simulink model "SimplePulseGenerator_4x4_HDL_IQ"  (R2019b)
settings: Solver=FixedStepDiscrete  StartTime=0.0  StopTime=inf  RelTol=1e-3
InitFcn:
  | %axis_example_init
  | nco_setup
  | load('iq_bus_obj.mat')
values from neighbouring files (symbols this model uses):
  Fo = 200.7e6    (= 200700000)    [model_init.m]
  Fs = 1/Ts    (= 512000000)    [model_init.m]
  incrScale = (2^N)/Fs    (= 3.2e-05)    [model_init.m]
  N = 14    [model_init.m]
  PRF_count_period = pspshared.libiio.aximm.write(                    'IPAddress',IPAddr,                    'AddressOffset',hex2dec('130'))    [SimplePulseGenerator_4x4_HDL_IQ_IIO_script.m]    (also in model_init.m = 1280)
  PulseWidth_count_width = PulseWidth*fpga_clk_rate/VectorSamplingFactor    (= 32)    [model_init.m]
libraries: hdlsllib x21, simulink x15, dsphdlsigops x4, simulink_need_slupdate x2, dspsrcs4 x1
(part 1 of 2)
Description:
  | HDL model for RFSoC ADC/DAC IQ 8x8 interfacing with the mixer enabled
  | 
  | This model contains demonstrates how to interface to all 8 ADC and 8 DAC
  | channels for the RFSoC.
  | 
  | Please ensure that you run the initialization script to set the correct PLL clock rates.
settings Model: DataTypeOverride=Off  Creator=mfornero  LastModifiedBy=tmealey
settings DataIOCC: SaveOutput=off  SaveTime=off  ReturnWorkspaceOutputs=off
settings OptimizationCC: BlockReduction=off  ConditionallyExecuteInputs=off  DefaultParameterBehavior=Inlined  LifeSpan=inf
settings DebuggingCC: AlgebraicLoopMsg=error  SingleTaskRateTransMsg=error  PregeneratedLibrarySubsystemCodeDiagnostic=none  StrictBusMsg=ErrorOnBusTreatedAsVector  SFUnexpectedBacktrackingDiag=warning  SFNoUnconditionalDefaultTransitionDiag=warning  SFExecutionAtInitializationDiag=none  ArithmeticOperatorsInVariantConditions=warning
settings HardwareCC: ProdBitPerPointer=32  ProdBitPerSizeT=32  ProdBitPerPtrDiffT=32  ProdLargestAtomicFloat=None  ProdIntDivRoundTo=Undefined  ProdEndianess=Unspecified  ProdWordSize=32  ProdHWDeviceType=ASIC/FPGA->ASIC/FPGA  ProdEqTarget=off
settings SFSimCC: SimUseLocalCustomCode=off  CustomCodeUndefinedFunction=UseInterfaceOnly
settings RTWCC: RTWUseLocalCustomCode=off
settings CodeAppCC: StateflowObjectComments=on
settings GRTTargetCC: TargetLangStandard=C89/C90 (ANSI)
settings ConfigComp: CovMetricSettings=dw  CovHtmlReporting=on  CovSaveCumulativeToWorkspaceVar=on  CovSaveSingleToWorkspaceVar=on  CovExternalEMLEnable=off

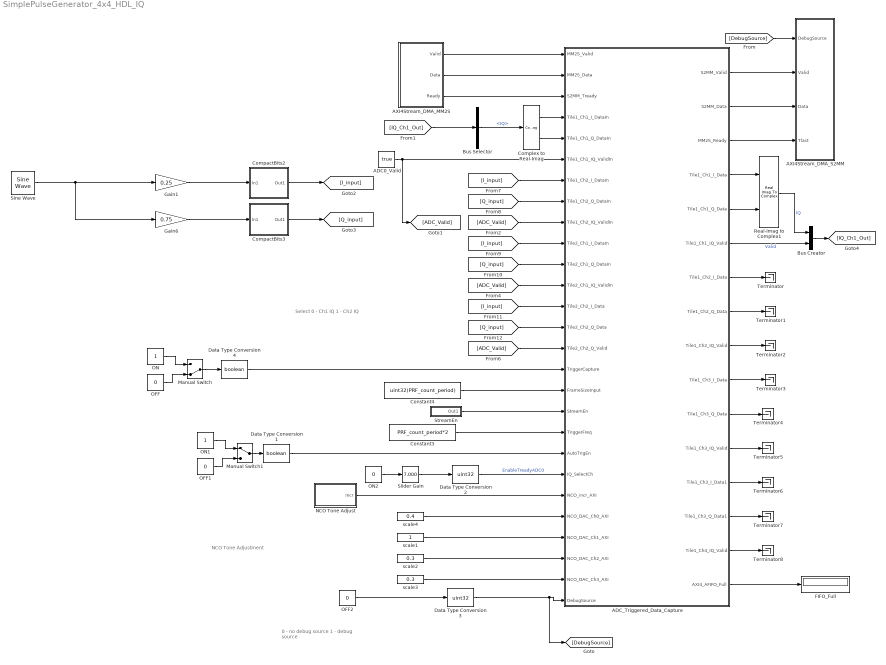
== system SimplePulseGenerator_4x4_HDL_IQ ==
  note: 0 - no debug source
      | 1 - debug source
  note: Select
      |
      | 0 - Ch1 IQ
      | 1 - Ch2 IQ
  note: NCO Tone Adjustment
  ADC0_Valid : Constant  Value=true  SampleTime=-1
  ADC_Triggered_Data_Capture : Subsystem  TreatAsAtomicUnit=on
  AXI4Stream_DMA_MM2S : Subsystem
  AXI4Stream_DMA_S2MM : Subsystem
  Bus Creator : BusCreator  Inputs=2
  Bus Selector : BusSelector  OutputSignals=IQ
  CompactBits2 : Subsystem
  CompactBits3 : Subsystem
  Complex to Real-Imag : ComplexToRealImag
  Constant3 : Constant  Value=PRF_count_period*2  OutDataTypeStr=uint32  SampleTime=-1
  Constant4 : Constant  Value=uint32(PRF_count_period)  SampleTime=-1
  Data Type Conversion1 : DataTypeConversion  OutDataTypeStr=boolean
  Data Type Conversion2 : DataTypeConversion  OutDataTypeStr=uint32
  Data Type Conversion3 : DataTypeConversion  OutDataTypeStr=uint32
  Data Type Conversion4 : DataTypeConversion  OutDataTypeStr=boolean
  FIFO_Full : Display
  Gain1 : Gain  Gain=0.25  OutDataTypeStr=Inherit: Same as input
  Gain6 : Gain  Gain=0.75  OutDataTypeStr=Inherit: Same as input
  Manual Switch : ManualSwitch  CurrentSetting=0
  Manual Switch1 : ManualSwitch
  NCO Tone Adjust : Subsystem
  OFF : Constant  Value=0  OutDataTypeStr=boolean  SampleTime=-1
  OFF1 : Constant  Value=0  OutDataTypeStr=boolean  SampleTime=-1
  OFF2 : Constant  Value=0  OutDataTypeStr=boolean  SampleTime=-1
  ON : Constant  OutDataTypeStr=boolean  SampleTime=-1
  ON1 : Constant  OutDataTypeStr=boolean  SampleTime=-1
  ON2 : Constant  Value=0  OutDataTypeStr=uint32  SampleTime=-1
  Real-Imag to Complex1 : RealImagToComplex
  Sine Wave : dspsrcs4/Sine Wave  Amplitude=1000  Frequency=0.1  Phase=0  SampleMode=Discrete  OutComplex=Real  CompMethod=Table lookup  TableSize=Speed  SampleTime=1/4  SamplesPerFrame=4  ResetState=Restart at time zero  OutputFrames=off  dataType=Fixed-point  wordLen=14  udDataType=sfix(16)  fracBitsMode=User-defined  numFracBits=0  OutDataTypeStr=fixdt(1,14,0)  LastOutDataTypeStr=fixdt(1,14,0)
  Slider Gain : simulink/Math Operations/Slider Gain  gain=7.000  low=0  high=7
  StreamEn : Subsystem
  Terminator{,1..8} (9 alike) : Terminator
  scale1 : Constant  OutDataTypeStr=fixdt(0,8,7)  SampleTime=-1
  scale2 : Constant  Value=0.3  OutDataTypeStr=fixdt(0,8,7)  SampleTime=-1
  scale3 : Constant  Value=0.3  OutDataTypeStr=fixdt(0,8,7)  SampleTime=-1
  scale4 : Constant  Value=0.4  OutDataTypeStr=fixdt(0,8,7)  SampleTime=-1
  wires:
  Data Type Conversion4/1 -> ADC_Triggered_Data_Capture/16(TriggerCapture)
  Constant4/1 -> ADC_Triggered_Data_Capture/17(FrameSizeInput)
  ADC0_Valid/1 -> [ADC_Valid], ADC_Triggered_Data_Capture/6(Tile1_Ch1_IQ_ValidIn)
  Manual Switch/1 -> Data Type Conversion4/1
  ON/1 -> Manual Switch/1
  OFF/1 -> Manual Switch/2
  scale4/1 -> ADC_Triggered_Data_Capture/23(NCO_DAC_Ch0_AXI)
  scale1/1 -> ADC_Triggered_Data_Capture/24(NCO_DAC_Ch1_AXI)
  scale2/1 -> ADC_Triggered_Data_Capture/25(NCO_DAC_Ch2_AXI)
  scale3/1 -> ADC_Triggered_Data_Capture/26(NCO_DAC_Ch3_AXI)
  StreamEn/1(Out1) -> ADC_Triggered_Data_Capture/18(StreamEn)
  Constant3/1 -> ADC_Triggered_Data_Capture/19(TriggerFreq)
  Data Type Conversion1/1 -> ADC_Triggered_Data_Capture/20(AutoTrigEn)
  OFF1/1 -> Manual Switch1/2
  ON1/1 -> Manual Switch1/1
  Manual Switch1/1 -> Data Type Conversion1/1
  ADC_Triggered_Data_Capture/16(AXI4_AFIFO_Full) -> FIFO_Full/1
  ADC_Triggered_Data_Capture/1(S2MM_Valid) -> AXI4Stream_DMA_S2MM/2(Valid)
  ADC_Triggered_Data_Capture/2(S2MM_Data) -> AXI4Stream_DMA_S2MM/3(Data)
  ADC_Triggered_Data_Capture/3(MM2S_Ready) -> AXI4Stream_DMA_S2MM/4(Tlast)
  AXI4Stream_DMA_MM2S/1(Valid) -> ADC_Triggered_Data_Capture/1(MM2S_Valid)
  AXI4Stream_DMA_MM2S/2(Data) -> ADC_Triggered_Data_Capture/2(MM2S_Data)
  AXI4Stream_DMA_MM2S/3(Ready) -> ADC_Triggered_Data_Capture/3(S2MM_Tready)
  ON2/1 -> Slider Gain/1
  Data Type Conversion2/1 -> ADC_Triggered_Data_Capture/21(IQ_SelectCh)  "EnableTreadyADC0"
  NCO Tone Adjust/1(Incr) -> ADC_Triggered_Data_Capture/22(NCO_incr_AXI)
  Slider Gain/1 -> Data Type Conversion2/1
  Sine Wave/1 -> Gain6/1, Gain1/1
  Gain1/1 -> CompactBits2/1(In1)
  Gain6/1 -> CompactBits3/1(In1)
  Data Type Conversion3/1 -> [DebugSource], ADC_Triggered_Data_Capture/27(DebugSource)
  OFF2/1 -> Data Type Conversion3/1
  [DebugSource] -> AXI4Stream_DMA_S2MM/1(DebugSource)
  [ADC_Valid] -> ADC_Triggered_Data_Capture/9(Tile1_Ch2_IQ_ValidIn)
  [ADC_Valid] -> ADC_Triggered_Data_Capture/12(Tile2_Ch1_IQ_ValidIn)
  [ADC_Valid] -> ADC_Triggered_Data_Capture/15(Tile2_Ch2_Q_Valid)
  CompactBits2/1(Out1) -> [I_input]
  CompactBits3/1(Out1) -> [Q_input]
  [I_input] -> ADC_Triggered_Data_Capture/7(Tile1_Ch2_I_DataIn)
  [Q_input] -> ADC_Triggered_Data_Capture/8(Tile1_Ch2_Q_DataIn)
  [I_input] -> ADC_Triggered_Data_Capture/10(Tile2_Ch1_I_DataIn)
  [Q_input] -> ADC_Triggered_Data_Capture/11(Tile2_Ch1_Q_DataIn)
  [I_input] -> ADC_Triggered_Data_Capture/13(Tile2_Ch2_I_Data)
  [Q_input] -> ADC_Triggered_Data_Capture/14(Tile2_Ch2_Q_Data)
  ADC_Triggered_Data_Capture/4(Tile1_Ch1_I_Data) -> Real-Imag to Complex1/1
  ADC_Triggered_Data_Capture/5(Tile1_Ch1_Q_Data) -> Real-Imag to Complex1/2
  Real-Imag to Complex1/1 -> Bus Creator/1  "IQ"
  ADC_Triggered_Data_Capture/6(Tile1_Ch1_IQ_Valid) -> Bus Creator/2  "Valid"
  Bus Creator/1 -> [IQ_Ch1_Out]
  ADC_Triggered_Data_Capture/7(Tile1_Ch2_I_Data) -> Terminator/1
  ADC_Triggered_Data_Capture/8(Tile1_Ch2_Q_Data) -> Terminator1/1
  ADC_Triggered_Data_Capture/9(Tile1_Ch2_IQ_Valid) -> Terminator2/1
  ADC_Triggered_Data_Capture/10(Tile1_Ch3_I_Data) -> Terminator3/1
  ADC_Triggered_Data_Capture/13(Tile1_Ch3_I_Data1) -> Terminator6/1
  ADC_Triggered_Data_Capture/11(Tile1_Ch3_Q_Data) -> Terminator4/1
  ADC_Triggered_Data_Capture/12(Tile1_Ch3_IQ_Valid) -> Terminator5/1
  ADC_Triggered_Data_Capture/14(Tile1_Ch3_Q_Data1) -> Terminator7/1
  ADC_Triggered_Data_Capture/15(Tile1_Ch4_IQ_Valid) -> Terminator8/1
  [IQ_Ch1_Out] -> Bus Selector/1
  Bus Selector/1 -> Complex to Real-Imag/1  "<IQ>"
  Complex to Real-Imag/1 -> ADC_Triggered_Data_Capture/4("Tile1_Ch1_I_DataIn ")
  Complex to Real-Imag/2 -> ADC_Triggered_Data_Capture/5(Tile1_Ch1_Q_DataIn)

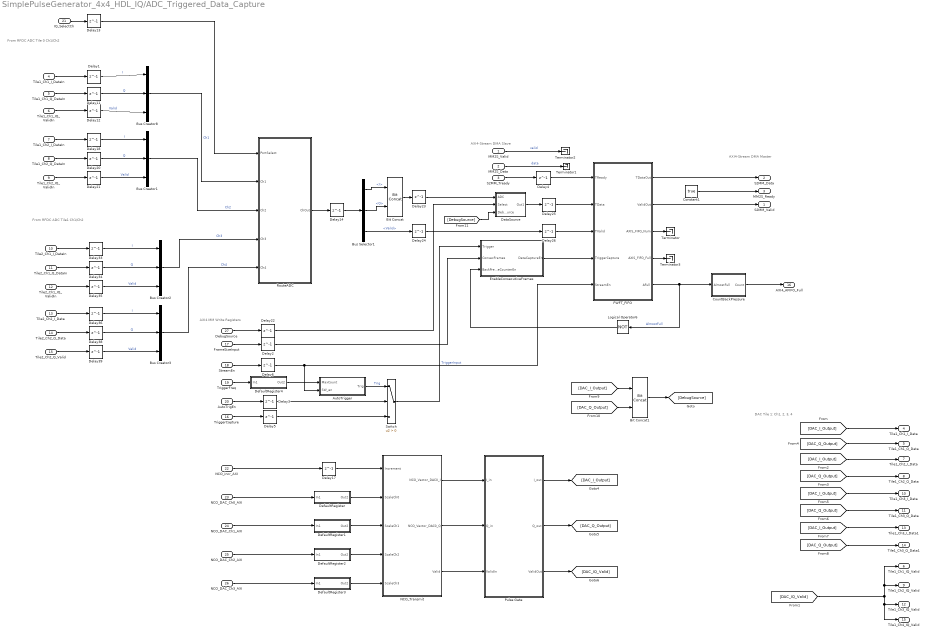
== system SimplePulseGenerator_4x4_HDL_IQ/ADC_Triggered_Data_Capture ==
  note: From RFDC ADC Tile1 Ch1/Ch2
  note: DAC Tile 1: Ch1, 2, 3, 4
  note: AXI4-Stream DMA Slave
  note: AXI4-Stream DMA Master
  note: AXI4 MM Write Registers
  note: From RFDC ADC Tile 0 Ch1/Ch2
  MM2S_Valid : Inport
  MM2S_Data : Inport  Port=2
  S2MM_Tready : Inport  Port=3
  "Tile1_Ch1_I_DataIn " : Inport  Port=4
  Tile1_Ch1_Q_DataIn : Inport  Port=5
  Tile1_Ch1_IQ_ValidIn : Inport  Port=6
  Tile1_Ch2_I_DataIn : Inport  Port=7
  Tile1_Ch2_Q_DataIn : Inport  Port=8
  Tile1_Ch2_IQ_ValidIn : Inport  Port=9
  Tile2_Ch1_I_DataIn : Inport  Port=10
  Tile2_Ch1_Q_DataIn : Inport  Port=11
  Tile2_Ch1_IQ_ValidIn : Inport  Port=12
  Tile2_Ch2_I_Data : Inport  Port=13
  Tile2_Ch2_Q_Data : Inport  Port=14
  Tile2_Ch2_Q_Valid : Inport  Port=15
  TriggerCapture : Inport  Port=16
  FrameSizeInput : Inport  Port=17
  StreamEn : Inport  Port=18
  TriggerFreq : Inport  Port=19
  AutoTrigEn : Inport  Port=20
  IQ_SelectCh : Inport  Port=21
  NCO_incr_AXI : Inport  Port=22
  NCO_DAC_Ch0_AXI : Inport  Port=23
  NCO_DAC_Ch1_AXI : Inport  Port=24
  NCO_DAC_Ch2_AXI : Inport  Port=25
  NCO_DAC_Ch3_AXI : Inport  Port=26
  DebugSource : Inport  Port=27
  AutoTrigger : Subsystem
  Bit Concat : hdlsllib/Logic and Bit Operations/Bit Concat  numInputs=2
      settings: SourceProductName=HDL Coder  SourceProductBaseCode=HD
  Bit Concat1 : hdlsllib/Logic and Bit Operations/Bit Concat  numInputs=2
      settings: SourceProductName=HDL Coder  SourceProductBaseCode=HD
  Bus Creator{1..3,8} (4 alike) : BusCreator  Inputs=3
  Bus Selector1 : BusSelector  OutputSignals=I,Q,Valid
  Constant1 : Constant  Value=true  OutDataTypeStr=boolean  SampleTime=-1
  CountBackPressure : Subsystem
  DataSource : Subsystem
  DefaultRegister : Subsystem
  DefaultRegister1 : Subsystem
  DefaultRegister2 : Subsystem
  DefaultRegister3 : Subsystem
  DefaultRegister4 : Subsystem
  Delay{1..6,11..14,17..18,20..26,33..36,38..39} (25 alike) : Delay  DelayLength=1
  EnableConsecutiveFrames : Subsystem
  FWFT_FIFO : Subsystem
  Logical Operator6 : Logic  Operator=NOT  IconShape=distinctive  AllPortsSameDT=off  OutDataTypeStr=boolean
  NCO_Transmit : Subsystem
  Pulse Gate : Subsystem
      settings: PortSchema="{\"entries\":[{\"content\":{\"sides\":[{\"content\":{\"connectorIds\":[\"In1\",\"In2\",\"In3\"]},\"type\":\"ConnectorPlacement.EquallySpacedRectSide\",\"uuid\":\"05cb44ea-d8d3-4536-b0b5-e0a95c346195\"},{\"content\":{\"connectorIds\":[\"Out1\",\"Out2\",\"Out3\"],\"side\":\"RIGHT\"},\"type\":\"ConnectorPlacement.EquallySpacedRectSide\",\"uuid\":\"95be599f-089a-458f-a20e-438c80ac73ea\"},{\"content\":{\"connectorIds\":[],\"side\":\"TOP\"},\"type\":\"ConnectorPlacement.EquallySpacedRectSide\",\"uuid\":\"53fe8b3e-6af9-4ca4-9119-803948436d03\"}]},\"type\":\"ConnectorPlacement.EquallySpacedConnector\",\"uuid\":\"f0d860a0-0621-4618-986c-a12bc105ad67\"}],\"packageUris\":[\"http://schema.mathworks.com/mf0/Connector/19700101\"],\"version\":\"1.0\"}"
  RouteADC : Subsystem
  Switch : Switch  Criteria=u2 > Threshold
  Terminator{,1..3} (4 alike) : Terminator
  S2MM_Valid : Outport  VectorParamsAs1DForOutWhenUnconnected=off
  S2MM_Data : Outport  Port=2  VectorParamsAs1DForOutWhenUnconnected=off
  MM2S_Ready : Outport  Port=3  VectorParamsAs1DForOutWhenUnconnected=off
  Tile1_Ch1_I_Data : Outport  Port=4  VectorParamsAs1DForOutWhenUnconnected=off
  Tile1_Ch1_Q_Data : Outport  Port=5  VectorParamsAs1DForOutWhenUnconnected=off
  Tile1_Ch1_IQ_Valid : Outport  Port=6  VectorParamsAs1DForOutWhenUnconnected=off
  Tile1_Ch2_I_Data : Outport  Port=7  VectorParamsAs1DForOutWhenUnconnected=off
  Tile1_Ch2_Q_Data : Outport  Port=8  VectorParamsAs1DForOutWhenUnconnected=off
  Tile1_Ch2_IQ_Valid : Outport  Port=9  VectorParamsAs1DForOutWhenUnconnected=off
  Tile1_Ch3_I_Data : Outport  Port=10  VectorParamsAs1DForOutWhenUnconnected=off
  Tile1_Ch3_Q_Data : Outport  Port=11  VectorParamsAs1DForOutWhenUnconnected=off
  Tile1_Ch3_IQ_Valid : Outport  Port=12  VectorParamsAs1DForOutWhenUnconnected=off
  Tile1_Ch3_I_Data1 : Outport  Port=13  VectorParamsAs1DForOutWhenUnconnected=off
  Tile1_Ch3_Q_Data1 : Outport  Port=14  VectorParamsAs1DForOutWhenUnconnected=off
  Tile1_Ch4_IQ_Valid : Outport  Port=15  VectorParamsAs1DForOutWhenUnconnected=off
  AXI4_AFIFO_Full : Outport  Port=16  VectorParamsAs1DForOutWhenUnconnected=off
  wires:
  MM2S_Valid/1 -> Terminator2/1  "valid"
  "Tile1_Ch1_I_DataIn "/1 -> Delay1/1
  MM2S_Data/1 -> Terminator1/1  "data"
  FWFT_FIFO/1(TDataOut) -> S2MM_Data/1
  FrameSizeInput/1 -> Delay2/1
  TriggerCapture/1 -> Delay5/1
  Delay5/1 -> Switch/3
  Delay2/1 -> EnableConsecutiveFrames/2(ConsecFrames)
  S2MM_Tready/1 -> Delay4/1
  Delay4/1 -> FWFT_FIFO/1(TReady)
  StreamEn/1 -> Delay6/1
  Delay6/1 -> AutoTrigger/2(SW_en), FWFT_FIFO/5(StreamEn)
  FWFT_FIFO/2(ValidOut) -> S2MM_Valid/1
  Constant1/1 -> MM2S_Ready/1
  NCO_incr_AXI/1 -> Delay17/1
  NCO_DAC_Ch0_AXI/1 -> DefaultRegister/1(In1)
  Delay17/1 -> NCO_Transmit/1(Increment)
  DefaultRegister/1(Out2) -> NCO_Transmit/2(ScaleCh0)
  DefaultRegister1/1(Out2) -> NCO_Transmit/3(ScaleCh1)
  DefaultRegister2/1(Out2) -> NCO_Transmit/4(ScaleCh2)
  DefaultRegister3/1(Out2) -> NCO_Transmit/5(ScaleCh3)
  NCO_DAC_Ch1_AXI/1 -> DefaultRegister1/1(In1)
  NCO_DAC_Ch2_AXI/1 -> DefaultRegister2/1(In1)
  NCO_DAC_Ch3_AXI/1 -> DefaultRegister3/1(In1)
  FWFT_FIFO/5(AFull) -> CountBackPressure/1(AlmostFull), Logical Operator6/1  "AlmostFull"
  Logical Operator6/1 -> EnableConsecutiveFrames/3(BackPressureCounterEn)
  EnableConsecutiveFrames/1(DataCaptureEn) -> FWFT_FIFO/4(TriggerCapture)
  Switch/1 -> EnableConsecutiveFrames/1(Trigger)  "TriggerInput"
  AutoTrigger/1(Trig) -> Switch/1  "Trig"
  TriggerFreq/1 -> DefaultRegister4/1(In1)
  DefaultRegister4/1(Out2) -> AutoTrigger/1(MaxCount)
  AutoTrigEn/1 -> Delay3/1
  Tile1_Ch1_IQ_ValidIn/1 -> Delay12/1
  Tile1_Ch1_Q_DataIn/1 -> Delay11/1
  Bus Selector1/3 -> Delay24/1  "<Valid>"
  IQ_SelectCh/1 -> Delay13/1
  Delay14/1 -> Bus Selector1/1
  Tile1_Ch2_I_DataIn/1 -> Delay18/1
  Tile1_Ch2_Q_DataIn/1 -> Delay20/1
  Tile1_Ch2_IQ_ValidIn/1 -> Delay21/1
  RouteADC/1(ChOut) -> Delay14/1
  Delay13/1 -> RouteADC/1(PortSelect)
  Bus Selector1/1 -> Bit Concat/1  "<I>"
  Bus Selector1/2 -> Bit Concat/2  "<Q>"
  Bit Concat/1 -> Delay23/1
  DebugSource/1 -> Delay22/1
  Delay24/1 -> Delay26/1
  Delay25/1 -> FWFT_FIFO/2(TData)
  Delay26/1 -> FWFT_FIFO/3(TValid)
  Delay23/1 -> DataSource/1(ADC)
  Delay22/1 -> DataSource/2(Select)
  DataSource/1(Out1) -> Delay25/1
  [DAC_IQ_Valid] -> Tile1_Ch1_IQ_Valid/1, Tile1_Ch2_IQ_Valid/1, Tile1_Ch4_IQ_Valid/1, Tile1_Ch3_IQ_Valid/1
  Tile2_Ch2_Q_Data/1 -> Delay38/1
  Delay39/1 -> Bus Creator3/3  "Valid"
  Tile2_Ch2_I_Data/1 -> Delay36/1
  Delay35/1 -> Bus Creator2/3  "Valid"
  Tile2_Ch1_Q_DataIn/1 -> Delay34/1
  Delay38/1 -> Bus Creator3/2  "Q"
  Tile2_Ch2_Q_Valid/1 -> Delay39/1
  Delay36/1 -> Bus Creator3/1  "I"
  Tile2_Ch1_IQ_ValidIn/1 -> Delay35/1
  Delay33/1 -> Bus Creator2/1  "I"
  Tile2_Ch1_I_DataIn/1 -> Delay33/1
  Delay34/1 -> Bus Creator2/2  "Q"
  Bus Creator2/1 -> RouteADC/4(Ch3)  "Ch3"
  Bus Creator8/1 -> RouteADC/2(Ch1)  "Ch1"
  FWFT_FIFO/3(AXIS_FIFO_Num) -> Terminator/1
  FWFT_FIFO/4(AXIS_FIFO_Full) -> Terminator3/1
  CountBackPressure/1(Count) -> AXI4_AFIFO_Full/1
  Delay11/1 -> Bus Creator8/2  "Q"
  Delay1/1 -> Bus Creator8/1  "I"
  Delay12/1 -> Bus Creator8/3  "Valid"
  Delay18/1 -> Bus Creator1/1  "I"
  Delay20/1 -> Bus Creator1/2  "Q"
  Delay21/1 -> Bus Creator1/3  "Valid"
  Bus Creator1/1 -> RouteADC/3(Ch2)  "Ch2"
  Bus Creator3/1 -> RouteADC/5(Ch4)  "Ch4"
  [DAC_I_Output] -> Tile1_Ch1_I_Data/1
  [DAC_I_Output] -> Tile1_Ch2_I_Data/1
  [DAC_Q_Output] -> Tile1_Ch1_Q_Data/1
  [DAC_Q_Output] -> Tile1_Ch2_Q_Data/1
  [DAC_I_Output] -> Tile1_Ch3_I_Data/1
  [DAC_Q_Output] -> Tile1_Ch3_Q_Data/1
  [DAC_Q_Output] -> Tile1_Ch3_Q_Data1/1
  [DAC_I_Output] -> Tile1_Ch3_I_Data1/1
  Delay3/1 -> Switch/2
  NCO_Transmit/3(Valid) -> Pulse Gate/3(ValidIn)
  NCO_Transmit/1(NCO_Vector_DAC0_I) -> Pulse Gate/1(I_in)
  NCO_Transmit/2(NCO_Vector_DAC0_Q) -> Pulse Gate/2(Q_in)
  Pulse Gate/1(I_out) -> [DAC_I_Output]
  Pulse Gate/2(Q_out) -> [DAC_Q_Output]
  Pulse Gate/3(ValidOut) -> [DAC_IQ_Valid]
  [DAC_I_Output] -> Bit Concat1/1
  [DAC_Q_Output] -> Bit Concat1/2
  Bit Concat1/1 -> [DebugSource]
  [DebugSource] -> DataSource/3(DebugSource)

== system SimplePulseGenerator_4x4_HDL_IQ/AXI4Stream_DMA_MM2S ==
  Constant : Constant  Value=true  SampleTime=-1
  S2MM DMA Ready : Constant  Value=true  SampleTime=-1
  TData : Constant  Value=0  OutDataTypeStr=fixdt(0,128,0)  SampleTime=-1
  Valid : Outport  VectorParamsAs1DForOutWhenUnconnected=off
  Data : Outport  Port=2  VectorParamsAs1DForOutWhenUnconnected=off
  Ready : Outport  Port=3  VectorParamsAs1DForOutWhenUnconnected=off
  wires:
  S2MM DMA Ready/1 -> Ready/1
  TData/1 -> Data/1
  Constant/1 -> Valid/1

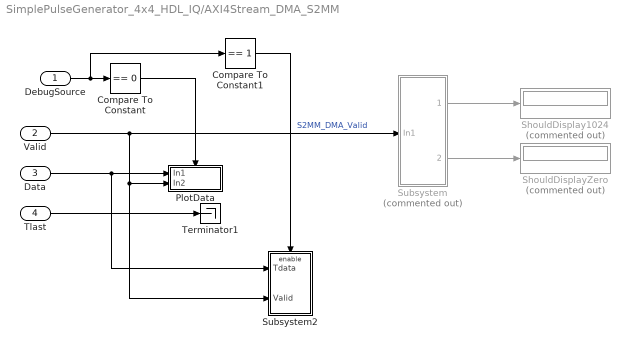
== system SimplePulseGenerator_4x4_HDL_IQ/AXI4Stream_DMA_S2MM ==
  DebugSource : Inport
  Valid : Inport  Port=2
  Data : Inport  Port=3
  Tlast : Inport  Port=4
  Compare To Constant : simulink/Logic and Bit Operations/Compare To Constant  relop===  const=0  OutDataTypeStr=boolean
  Compare To Constant1 : simulink/Logic and Bit Operations/Compare To Constant  relop===  const=1  OutDataTypeStr=boolean
  PlotData : Subsystem
  ShouldDisplay1024 : Display  Commented=on
  ShouldDisplayZero : Display  Commented=on
  Subsystem : Subsystem  Commented=on
  Subsystem2 : Subsystem
  Terminator1 : Terminator
  wires:
  Tlast/1 -> Terminator1/1
  Subsystem/1(Out1) -> ShouldDisplay1024/1
  Subsystem/2(Out2) -> ShouldDisplayZero/1
  Valid/1 -> Subsystem2/2(Valid), PlotData/2(In2), Subsystem/1(In1)  "S2MM_DMA_Valid"
  Data/1 -> Subsystem2/1(Tdata), PlotData/1(In1)
  DebugSource/1 -> Compare To Constant1/1, Compare To Constant/1
  Compare To Constant/1 -> PlotData/Enable
  Compare To Constant1/1 -> Subsystem2/Enable

== system SimplePulseGenerator_4x4_HDL_IQ/CompactBits2 ==
  In1 : Inport
  Bit Concat : hdlsllib/Logic and Bit Operations/Bit Concat  numInputs=4
      settings: SourceProductName=HDL Coder  SourceProductBaseCode=HD
  Data Type Conversion{,1..3} (4 alike) : DataTypeConversion  OutDataTypeStr=fixdt(1,16,0)  ConvertRealWorld=Stored Integer (SI)
  Demux : Demux
  Out1 : Outport  VectorParamsAs1DForOutWhenUnconnected=off
  wires:
  Demux/4 -> Data Type Conversion3/1
  Demux/1 -> Data Type Conversion/1
  Data Type Conversion3/1 -> Bit Concat/1
  Demux/2 -> Data Type Conversion1/1
  Data Type Conversion2/1 -> Bit Concat/2
  Bit Concat/1 -> Out1/1
  Data Type Conversion/1 -> Bit Concat/4
  Data Type Conversion1/1 -> Bit Concat/3
  Demux/3 -> Data Type Conversion2/1
  In1/1 -> Demux/1

== system SimplePulseGenerator_4x4_HDL_IQ/CompactBits3 ==
  In1 : Inport
  Bit Concat : hdlsllib/Logic and Bit Operations/Bit Concat  numInputs=4
      settings: SourceProductName=HDL Coder  SourceProductBaseCode=HD
  Data Type Conversion{,1..3} (4 alike) : DataTypeConversion  OutDataTypeStr=fixdt(1,16,0)  ConvertRealWorld=Stored Integer (SI)
  Demux : Demux
  Out1 : Outport  VectorParamsAs1DForOutWhenUnconnected=off
  wires:
  In1/1 -> Demux/1
  Demux/3 -> Data Type Conversion2/1
  Data Type Conversion1/1 -> Bit Concat/3
  Data Type Conversion/1 -> Bit Concat/4
  Bit Concat/1 -> Out1/1
  Data Type Conversion2/1 -> Bit Concat/2
  Demux/2 -> Data Type Conversion1/1
  Data Type Conversion3/1 -> Bit Concat/1
  Demux/1 -> Data Type Conversion/1
  Demux/4 -> Data Type Conversion3/1

== system SimplePulseGenerator_4x4_HDL_IQ/NCO Tone Adjust ==
  Constant2 : Constant  SampleTime=-1
  Data Type Conversion : DataTypeConversion  OutDataTypeStr=uint16
  Freq (MHz) : simulink/Math Operations/Slider Gain  gain=57.5  low=0  high=250
  Gain : Gain  Gain=1e6
  Gain1 : Gain  Gain=incrScale
  Incr : Outport  VectorParamsAs1DForOutWhenUnconnected=off
  wires:
  Freq (MHz)/1 -> Gain/1
  Constant2/1 -> Freq (MHz)/1
  Data Type Conversion/1 -> Incr/1
  Gain1/1 -> Data Type Conversion/1
  Gain/1 -> Gain1/1

== system SimplePulseGenerator_4x4_HDL_IQ/StreamEn ==
  Data Type Conversion1 : DataTypeConversion  OutDataTypeStr=boolean
  Manual Switch1 : ManualSwitch
  OFF1 : Constant  Value=0  OutDataTypeStr=boolean  SampleTime=-1
  ON1 : Constant  OutDataTypeStr=boolean  SampleTime=-1
  Out1 : Outport  VectorParamsAs1DForOutWhenUnconnected=off
  wires:
  Data Type Conversion1/1 -> Out1/1
  OFF1/1 -> Manual Switch1/2
  ON1/1 -> Manual Switch1/1
  Manual Switch1/1 -> Data Type Conversion1/1

== system SimplePulseGenerator_4x4_HDL_IQ/ADC_Triggered_Data_Capture/AutoTrigger ==
  MaxCount : Inport
  SW_en : Inport  Port=2
  DataPushFrequency : hdlsllib/Sources/HDL Counter  CountType=Free running  CountInit=0  CountStep=1  CountMax=25  CountFromType=Initial value  CountFrom=0  CountResetPort=on  CountLoadPort=off  CountEnbPort=on  CountDirPort=off  CountDataType=Unsigned  CountWordLen=32  CountFracLen=0  CountSampTime=1
      settings: SourceProductBaseCode=HD
  Detect Increase : simulink/Logic and Bit Operations/Detect Increase  vinit=0.0  OutDataTypeStr=boolean
  Relational Operator : RelationalOperator  Operator===  OutDataTypeStr=boolean  RndMeth=Simplest
  Trig : Outport  VectorParamsAs1DForOutWhenUnconnected=off
  wires:
  Relational Operator/1 -> DataPushFrequency/1, Detect Increase/1
  DataPushFrequency/1 -> Relational Operator/2  "DataPushFrequencyCount"
  Detect Increase/1 -> Trig/1
  SW_en/1 -> DataPushFrequency/2
  MaxCount/1 -> Relational Operator/1

== system SimplePulseGenerator_4x4_HDL_IQ/ADC_Triggered_Data_Capture/CountBackPressure ==
  AlmostFull : Inport
  Add : Sum  AccumDataTypeStr=uint32
  Data Type Conversion : DataTypeConversion  OutDataTypeStr=uint32
  Delay16 : Delay  DelayLength=1
  Count : Outport  VectorParamsAs1DForOutWhenUnconnected=off
  wires:
  Delay16/1 -> Count/1, Add/2
  Add/1 -> Delay16/1
  Data Type Conversion/1 -> Add/1
  AlmostFull/1 -> Data Type Conversion/1

== system SimplePulseGenerator_4x4_HDL_IQ/ADC_Triggered_Data_Capture/DataSource ==
  ADC : Inport
  Select : Inport  Port=2
  DebugSource : Inport  Port=3
  Multiport Switch : MultiPortSwitch  DataPortOrder=Zero-based contiguous  Inputs=2  DataPortForDefault=Additional data port  DiagnosticForDefault=Warning  zeroidx=on
  Out1 : Outport  VectorParamsAs1DForOutWhenUnconnected=off
  wires:
  ADC/1 -> Multiport Switch/2, Multiport Switch/4
  Select/1 -> Multiport Switch/1
  DebugSource/1 -> Multiport Switch/3
  Multiport Switch/1 -> Out1/1

== system SimplePulseGenerator_4x4_HDL_IQ/ADC_Triggered_Data_Capture/DefaultRegister ==
  note: Give it default non-zero value at start-up time
  In1 : Inport
  Compare To Zero : simulink/Logic and Bit Operations/Compare To Zero  relop===  OutDataTypeStr=boolean
  Constant5 : Constant  Value=0.0625  OutDataTypeStr=fixdt(0,4,4)  SampleTime=-1
  Delay1 : Delay  DelayLength=1
  Switch2 : Switch  Criteria=u2 > Threshold
  Out2 : Outport  VectorParamsAs1DForOutWhenUnconnected=off
  wires:
  In1/1 -> Delay1/1
  Constant5/1 -> Switch2/1
  Delay1/1 -> Switch2/3, Compare To Zero/1
  Switch2/1 -> Out2/1
  Compare To Zero/1 -> Switch2/2

== system SimplePulseGenerator_4x4_HDL_IQ/ADC_Triggered_Data_Capture/DefaultRegister1 ==
  note: Give it default non-zero value at start-up time
  In1 : Inport
  Compare To Zero : simulink/Logic and Bit Operations/Compare To Zero  relop===  OutDataTypeStr=boolean
  Constant5 : Constant  Value=0.3  OutDataTypeStr=fixdt(0,4,4)  SampleTime=-1
  Delay1 : Delay  DelayLength=1
  Switch2 : Switch  Criteria=u2 > Threshold
  Out2 : Outport  VectorParamsAs1DForOutWhenUnconnected=off
  wires:
  Compare To Zero/1 -> Switch2/2
  Switch2/1 -> Out2/1
  Delay1/1 -> Compare To Zero/1, Switch2/3
  Constant5/1 -> Switch2/1
  In1/1 -> Delay1/1

== system SimplePulseGenerator_4x4_HDL_IQ/ADC_Triggered_Data_Capture/DefaultRegister2 ==
  note: Give it default non-zero value at start-up time
  In1 : Inport
  Compare To Zero : simulink/Logic and Bit Operations/Compare To Zero  relop===  OutDataTypeStr=boolean
  Constant5 : Constant  Value=0.3  OutDataTypeStr=fixdt(0,4,4)  SampleTime=-1
  Delay1 : Delay  DelayLength=1
  Switch2 : Switch  Criteria=u2 > Threshold
  Out2 : Outport  VectorParamsAs1DForOutWhenUnconnected=off
  wires:
  In1/1 -> Delay1/1
  Constant5/1 -> Switch2/1
  Delay1/1 -> Switch2/3, Compare To Zero/1
  Switch2/1 -> Out2/1
  Compare To Zero/1 -> Switch2/2

== system SimplePulseGenerator_4x4_HDL_IQ/ADC_Triggered_Data_Capture/DefaultRegister3 ==
  note: Give it default non-zero value at start-up time
  In1 : Inport
  Compare To Zero : simulink/Logic and Bit Operations/Compare To Zero  relop===  OutDataTypeStr=boolean
  Constant5 : Constant  Value=0.3  OutDataTypeStr=fixdt(0,4,4)  SampleTime=-1
  Delay1 : Delay  DelayLength=1
  Switch2 : Switch  Criteria=u2 > Threshold
  Out2 : Outport  VectorParamsAs1DForOutWhenUnconnected=off
  wires:
  Compare To Zero/1 -> Switch2/2
  Switch2/1 -> Out2/1
  Delay1/1 -> Compare To Zero/1, Switch2/3
  Constant5/1 -> Switch2/1
  In1/1 -> Delay1/1

== system SimplePulseGenerator_4x4_HDL_IQ/ADC_Triggered_Data_Capture/DefaultRegister4 ==
  note: Trigger every 0.5 sec by default
  In1 : Inport
  Compare To Zero : simulink/Logic and Bit Operations/Compare To Zero  relop===  OutDataTypeStr=boolean
  Constant5 : Constant  Value=62500000  OutDataTypeStr=uint32  SampleTime=-1
  Delay1 : Delay  DelayLength=1
  Switch2 : Switch  Criteria=u2 > Threshold
  Out2 : Outport  VectorParamsAs1DForOutWhenUnconnected=off
  wires:
  In1/1 -> Delay1/1
  Constant5/1 -> Switch2/1
  Delay1/1 -> Switch2/3, Compare To Zero/1
  Switch2/1 -> Out2/1
  Compare To Zero/1 -> Switch2/2

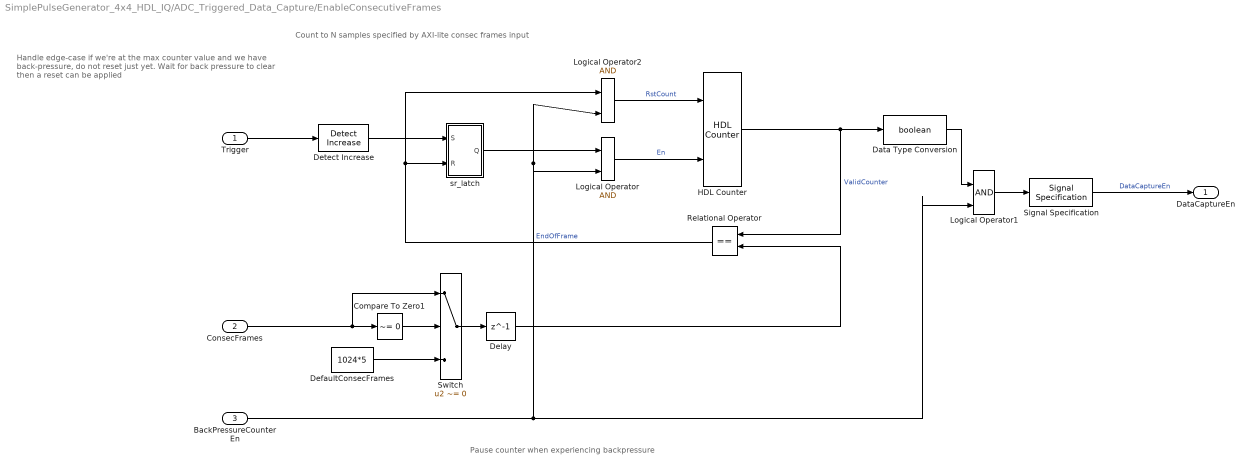
== system SimplePulseGenerator_4x4_HDL_IQ/ADC_Triggered_Data_Capture/EnableConsecutiveFrames ==
  note: Pause counter when experiencing backpressure
  note: Handle edge-case if we're at the
      | max counter value and we have back-pressure, do not reset
      | just yet. Wait for back pressure to clear then a reset can be applied
  note: Count to N samples specified by AXI-lite consec frames input
  Trigger : Inport
  ConsecFrames : Inport  Port=2
  BackPressureCounterEn : Inport  Port=3
  Compare To Zero1 : simulink/Logic and Bit Operations/Compare To Zero  relop=~=  OutDataTypeStr=boolean
  Data Type Conversion : DataTypeConversion  OutDataTypeStr=boolean
  DefaultConsecFrames : Constant  Value=1024*5  OutDataTypeStr=uint32  SampleTime=-1
  Delay : Delay  DelayLength=1
  Detect Increase : simulink/Logic and Bit Operations/Detect Increase  vinit=0.0  OutDataTypeStr=boolean
  HDL Counter : hdlsllib/Sources/HDL Counter  CountType=Free running  CountInit=0  CountStep=1  CountMax=25  CountFromType=Initial value  CountFrom=0  CountResetPort=on  CountLoadPort=off  CountEnbPort=on  CountDirPort=off  CountDataType=Unsigned  CountWordLen=32  CountFracLen=0  CountSampTime=1
      settings: SourceProductBaseCode=HD
  Logical Operator : Logic  IconShape=distinctive  AllPortsSameDT=off  OutDataTypeStr=boolean
  Logical Operator1 : Logic  IconShape=distinctive  AllPortsSameDT=off  OutDataTypeStr=boolean
  Logical Operator2 : Logic  IconShape=distinctive  AllPortsSameDT=off  OutDataTypeStr=boolean
  Relational Operator : RelationalOperator  Operator===  OutDataTypeStr=boolean  RndMeth=Simplest
  Signal Specification : SignalSpecification  OutDataTypeStr=boolean  Dimensions=1
  Switch : Switch  Criteria=u2 ~= 0
  sr_latch : Subsystem
  DataCaptureEn : Outport  VectorParamsAs1DForOutWhenUnconnected=off
  wires:
  Signal Specification/1 -> DataCaptureEn/1  "DataCaptureEn"
  Detect Increase/1 -> sr_latch/1(S)
  sr_latch/1(Q) -> Logical Operator/1
  HDL Counter/1 -> Relational Operator/1, Data Type Conversion/1  "ValidCounter"
  Trigger/1 -> Detect Increase/1
  ConsecFrames/1 -> Switch/1, Compare To Zero1/1
  Compare To Zero1/1 -> Switch/2
  Switch/1 -> Delay/1
  DefaultConsecFrames/1 -> Switch/3
  Logical Operator/1 -> HDL Counter/2  "En"
  Data Type Conversion/1 -> Logical Operator1/1
  Logical Operator1/1 -> Signal Specification/1
  Relational Operator/1 -> Logical Operator2/1, sr_latch/2(R)  "EndOfFrame"
  BackPressureCounterEn/1 -> Logical Operator1/2, Logical Operator2/2, Logical Operator/2
  Logical Operator2/1 -> HDL Counter/1  "RstCount"
  Delay/1 -> Relational Operator/2

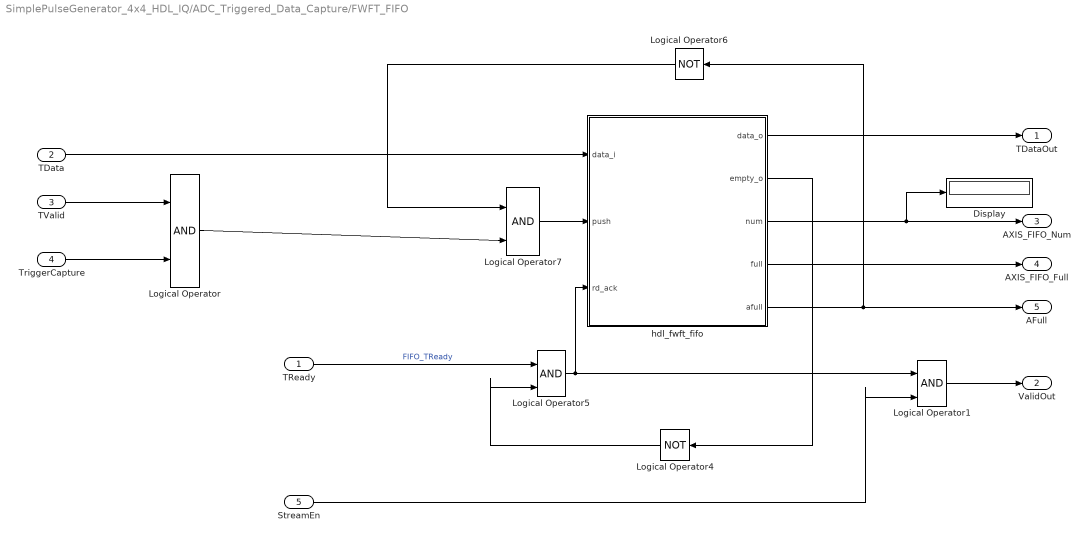
== system SimplePulseGenerator_4x4_HDL_IQ/ADC_Triggered_Data_Capture/FWFT_FIFO ==
  TReady : Inport
  TData : Inport  Port=2
  TValid : Inport  Port=3
  TriggerCapture : Inport  Port=4
  StreamEn : Inport  Port=5
  Display : Display
  Logical Operator : Logic  AllPortsSameDT=off  OutDataTypeStr=boolean
  Logical Operator1 : Logic  IconShape=distinctive  AllPortsSameDT=off  OutDataTypeStr=boolean
  Logical Operator4 : Logic  Operator=NOT  IconShape=distinctive  AllPortsSameDT=off  OutDataTypeStr=boolean
  Logical Operator5 : Logic  IconShape=distinctive  AllPortsSameDT=off  OutDataTypeStr=boolean
  Logical Operator6 : Logic  Operator=NOT  IconShape=distinctive  AllPortsSameDT=off  OutDataTypeStr=boolean
  Logical Operator7 : Logic  IconShape=distinctive  AllPortsSameDT=off  OutDataTypeStr=boolean
  hdl_fwft_fifo : Subsystem  mask{FIFO_DEPTH=1024*10, AFULL_THRESH=10}
      mask prompts: FIFO_DEPTH "FIFO Depth"; AFULL_THRESH "Almost Full Threshold"
      mask init:
      | FIFO_CNT_BITS=ceil(log2(FIFO_DEPTH+1+3));
  TDataOut : Outport  VectorParamsAs1DForOutWhenUnconnected=off
  ValidOut : Outport  Port=2  VectorParamsAs1DForOutWhenUnconnected=off
  AXIS_FIFO_Num : Outport  Port=3  VectorParamsAs1DForOutWhenUnconnected=off
  AXIS_FIFO_Full : Outport  Port=4  VectorParamsAs1DForOutWhenUnconnected=off
  AFull : Outport  Port=5  VectorParamsAs1DForOutWhenUnconnected=off
  wires:
  TValid/1 -> Logical Operator/1
  Logical Operator6/1 -> Logical Operator7/1
  Logical Operator4/1 -> Logical Operator5/2
  Logical Operator5/1 -> Logical Operator1/1, hdl_fwft_fifo/3(rd_ack)
  Logical Operator7/1 -> hdl_fwft_fifo/2(push)
  TReady/1 -> Logical Operator5/1  "FIFO_TReady"
  hdl_fwft_fifo/5(afull) -> AFull/1, Logical Operator6/1
  hdl_fwft_fifo/4(full) -> AXIS_FIFO_Full/1
  Logical Operator/1 -> Logical Operator7/2
  hdl_fwft_fifo/2(empty_o) -> Logical Operator4/1
  hdl_fwft_fifo/3(num) -> Display/1, AXIS_FIFO_Num/1
  TriggerCapture/1 -> Logical Operator/2
  TData/1 -> hdl_fwft_fifo/1(data_i)
  hdl_fwft_fifo/1(data_o) -> TDataOut/1
  Logical Operator1/1 -> ValidOut/1
  StreamEn/1 -> Logical Operator1/2

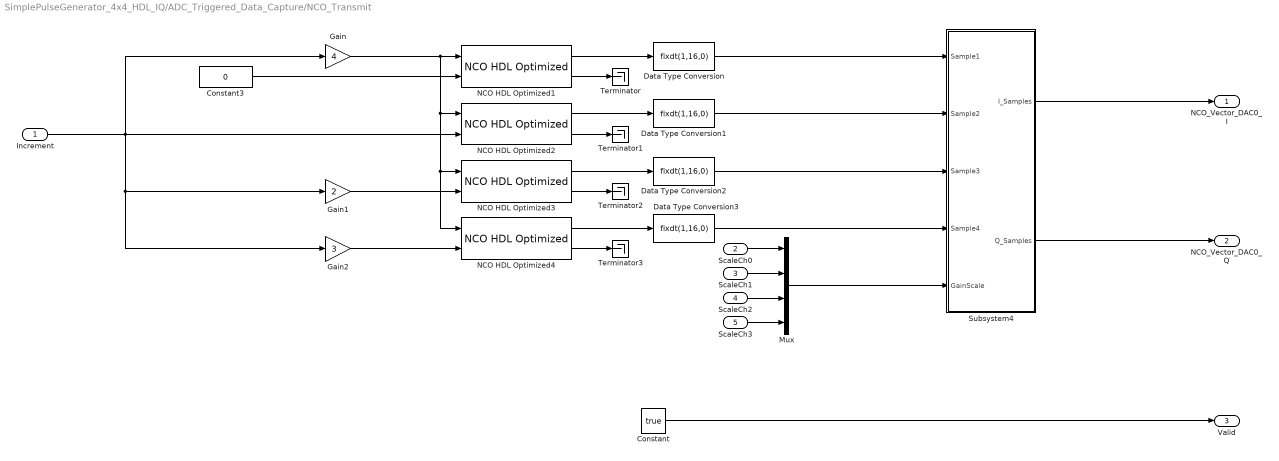
== system SimplePulseGenerator_4x4_HDL_IQ/ADC_Triggered_Data_Capture/NCO_Transmit ==
  Increment : Inport
  ScaleCh0 : Inport  Port=2
  ScaleCh1 : Inport  Port=3
  ScaleCh2 : Inport  Port=4
  ScaleCh3 : Inport  Port=5
  Constant : Constant  Value=true  SampleTime=-1
  Constant3 : Constant  Value=0  OutDataTypeStr=uint16  SampleTime=-1
  Data Type Conversion{,1..3} (4 alike) : DataTypeConversion  OutDataTypeStr=fixdt(1,16,0)  ConvertRealWorld=Stored Integer (SI)
  Gain : Gain  Gain=4  OutDataTypeStr=uint16  ParamDataTypeStr=Inherit: Same as input
  Gain1 : Gain  Gain=2  OutDataTypeStr=Inherit: Same as input
  Gain2 : Gain  Gain=3  OutDataTypeStr=Inherit: Same as input
  Mux : Mux
  NCO HDL Optimized{1..4} (4 alike) : dsphdlsigops/NCO HDL Optimized  PhaseIncrementSource=Input port  PhaseIncrement=round(Fo*(2^N)/Fs)  PhaseOffsetSource=Input port  PhaseOffset=0  DitherSource=Property  NumDitherBits=4  PhaseQuantization=off  NumQuantizerAccumulatorBits=12  LUTCompress=on  ResetAction=off  ValidInputPort=off  Waveform=Complex exponential  PhasePort=off  SimulateUsing=Code generation  AccumulatorWL=N  OutputDataType=Binary point scaling  OutputWL=14  OutputFL=12
      settings: SourceProductName=DSP System Toolbox  SourceProductBaseCode=DS
  Subsystem4 : Subsystem
  Terminator{,1..3} (4 alike) : Terminator
  NCO_Vector_DAC0_I : Outport  VectorParamsAs1DForOutWhenUnconnected=off
  NCO_Vector_DAC0_Q : Outport  Port=2  VectorParamsAs1DForOutWhenUnconnected=off
  Valid : Outport  Port=3  VectorParamsAs1DForOutWhenUnconnected=off
  wires:
  Gain/1 -> NCO HDL Optimized1/1, NCO HDL Optimized2/1, NCO HDL Optimized4/1, NCO HDL Optimized3/1
  Constant3/1 -> NCO HDL Optimized1/2
  Increment/1 -> Gain/1, NCO HDL Optimized2/2, Gain2/1, Gain1/1
  Gain2/1 -> NCO HDL Optimized4/2
  Gain1/1 -> NCO HDL Optimized3/2
  Constant/1 -> Valid/1
  NCO HDL Optimized1/1 -> Data Type Conversion/1
  NCO HDL Optimized2/1 -> Data Type Conversion1/1
  NCO HDL Optimized3/1 -> Data Type Conversion2/1
  NCO HDL Optimized4/1 -> Data Type Conversion3/1
  NCO HDL Optimized1/2 -> Terminator/1
  NCO HDL Optimized2/2 -> Terminator1/1
  NCO HDL Optimized3/2 -> Terminator2/1
  NCO HDL Optimized4/2 -> Terminator3/1
  Data Type Conversion/1 -> Subsystem4/1(Sample1)
  Data Type Conversion1/1 -> Subsystem4/2(Sample2)
  Data Type Conversion2/1 -> Subsystem4/3(Sample3)
  Data Type Conversion3/1 -> Subsystem4/4(Sample4)
  ScaleCh0/1 -> Mux/1
  ScaleCh1/1 -> Mux/2
  ScaleCh2/1 -> Mux/3
  ScaleCh3/1 -> Mux/4
  Mux/1 -> Subsystem4/5(GainScale)
  Subsystem4/1(I_Samples) -> NCO_Vector_DAC0_I/1
  Subsystem4/2(Q_Samples) -> NCO_Vector_DAC0_Q/1

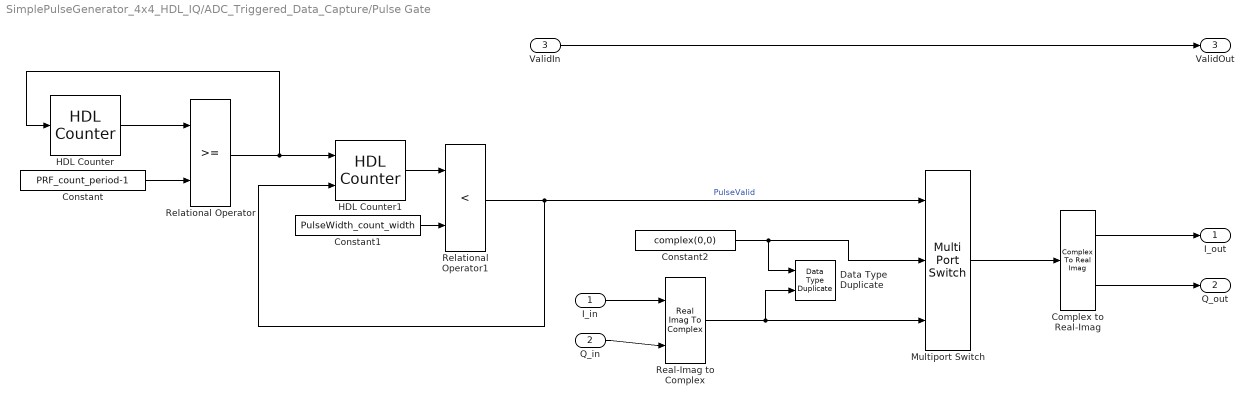
== system SimplePulseGenerator_4x4_HDL_IQ/ADC_Triggered_Data_Capture/Pulse Gate ==
  I_in : Inport
  Q_in : Inport  Port=2
  ValidIn : Inport  Port=3
  Complex to Real-Imag : ComplexToRealImag
  Constant : Constant  Value=PRF_count_period-1  OutDataTypeStr=uint32  SampleTime=-1
  Constant1 : Constant  Value=PulseWidth_count_width  OutDataTypeStr=uint32  SampleTime=-1
  Constant2 : Constant  Value=complex(0,0)  OutDataTypeStr=Inherit: Inherit via back propagation  SampleTime=-1
  Data Type Duplicate : DataTypeDuplicate
  HDL Counter : hdlsllib/Sources/HDL Counter  CountType=Free running  CountInit=0  CountStep=1  CountMax=25  CountFromType=Initial value  CountFrom=0  CountResetPort=on  CountLoadPort=off  CountEnbPort=off  CountDirPort=off  CountDataType=Unsigned  CountWordLen=32  CountFracLen=0  CountSampTime=-1
      settings: SourceProductName=Simulink
  HDL Counter1 : hdlsllib/Sources/HDL Counter  CountType=Free running  CountInit=0  CountStep=1  CountMax=25  CountFromType=Initial value  CountFrom=0  CountResetPort=on  CountLoadPort=off  CountEnbPort=on  CountDirPort=off  CountDataType=Unsigned  CountWordLen=32  CountFracLen=0  CountSampTime=-1
      settings: SourceProductName=Simulink
  Multiport Switch : MultiPortSwitch  DataPortOrder=Zero-based contiguous  Inputs=2  zeroidx=on
  Real-Imag to Complex : RealImagToComplex
  Relational Operator : RelationalOperator  OutDataTypeStr=boolean  RndMeth=Simplest
  Relational Operator1 : RelationalOperator  Operator=<  OutDataTypeStr=boolean  RndMeth=Simplest
  I_out : Outport
  Q_out : Outport  Port=2
  ValidOut : Outport  Port=3
  wires:
  Q_in/1 -> Real-Imag to Complex/2
  I_in/1 -> Real-Imag to Complex/1
  Complex to Real-Imag/1 -> I_out/1
  Complex to Real-Imag/2 -> Q_out/1
  HDL Counter/1 -> Relational Operator/1
  Constant/1 -> Relational Operator/2
  Relational Operator/1 -> HDL Counter1/1, HDL Counter/1
  HDL Counter1/1 -> Relational Operator1/1
  Constant1/1 -> Relational Operator1/2
  Relational Operator1/1 -> HDL Counter1/2, Multiport Switch/1  "PulseValid"
  Real-Imag to Complex/1 -> Data Type Duplicate/2, Multiport Switch/3
  Constant2/1 -> Data Type Duplicate/1, Multiport Switch/2
  Multiport Switch/1 -> Complex to Real-Imag/1
  ValidIn/1 -> ValidOut/1

== system SimplePulseGenerator_4x4_HDL_IQ/ADC_Triggered_Data_Capture/RouteADC ==
  PortSelect : Inport
  Ch1 : Inport  Port=2
  Ch2 : Inport  Port=3
  Ch3 : Inport  Port=4
  Ch4 : Inport  Port=5
  Multiport Switch : MultiPortSwitch  DataPortOrder=Zero-based contiguous  Inputs=4  DataPortForDefault=Additional data port  DiagnosticForDefault=Warning  zeroidx=on
  ChOut : Outport  VectorParamsAs1DForOutWhenUnconnected=off
  wires:
  PortSelect/1 -> Multiport Switch/1
  Ch1/1 -> Multiport Switch/6, Multiport Switch/2
  Multiport Switch/1 -> ChOut/1
  Ch2/1 -> Multiport Switch/3
  Ch3/1 -> Multiport Switch/4
  Ch4/1 -> Multiport Switch/5

== system SimplePulseGenerator_4x4_HDL_IQ/AXI4Stream_DMA_S2MM/PlotData ==
  In1 : Inport
  In2 : Inport  Port=2
  Enable : EnablePort
  Bit Slice1 : hdlsllib/Logic and Bit Operations/Bit Slice  lidx=63  ridx=0
  Bit Slice4 : hdlsllib/Logic and Bit Operations/Bit Slice  lidx=127  ridx=64
  Real-Imag to Complex : RealImagToComplex
  Subsystem : Subsystem
  Subsystem1 : Subsystem
  Time Scope : Scope  NumInputPorts=2
  wires:
  In1/1 -> Bit Slice4/1, Bit Slice1/1
  In2/1 -> Time Scope/2
  Bit Slice4/1 -> Subsystem/1(In1)
  Bit Slice1/1 -> Subsystem1/1(In1)
  Subsystem/1(Out1) -> Real-Imag to Complex/1
  Subsystem1/1(Out1) -> Real-Imag to Complex/2
  Real-Imag to Complex/1 -> Time Scope/1

== system SimplePulseGenerator_4x4_HDL_IQ/AXI4Stream_DMA_S2MM/Subsystem ==
  In1 : Inport
  Add : Sum  AccumDataTypeStr=uint32
  Constant3 : Constant  Value=1024  OutDataTypeStr=uint32  SampleTime=-1
  Data Type Conversion1 : DataTypeConversion  OutDataTypeStr=uint32
  Delay : Delay  DelayLength=1
  Mod : Math  Operator=mod  SaturateOnIntegerOverflow=on
  Out1 : Outport  VectorParamsAs1DForOutWhenUnconnected=off
  Out2 : Outport  Port=2  VectorParamsAs1DForOutWhenUnconnected=off
  wires:
  Mod/1 -> Out2/1
  Delay/1 -> Out1/1, Mod/1, Add/2
  Data Type Conversion1/1 -> Add/1
  In1/1 -> Data Type Conversion1/1
  Constant3/1 -> Mod/2
  Add/1 -> Delay/1

== system SimplePulseGenerator_4x4_HDL_IQ/AXI4Stream_DMA_S2MM/Subsystem2 ==
  Tdata : Inport
  Valid : Inport  Port=2
  Enable : EnablePort
  Subsystem1 : Subsystem  mask{samplesPerClock=4, complexSamples=on, reqBitWidth=0}
      mask prompts: samplesPerClock "Samples per clock"; complexSamples "Complex Samples"
      mask init:
      | if complexSamples
      |     input_length = samplesPerClock*2;
      | else
      |     input_length = samplesPerClock;
      | end
      | reqBitWidth = input_length*16;
      mask Display:
      | SamplesPerClock = get(gcbh,'SamplesPerClock')
      | ComplexSamples = get(gcbh,'ComplexSamples')
      | NumSample = str2num(SamplesPerClock);
      | if strcmp(ComplexSamples,'on')
      |     BitWidth = NumSample*2*16
      |     msg_bottom = 'Complex';
      |     label_out = sprintf('[%dx16-bit]',NumSample);
      | 
      | else
      |     BitWidth = NumSample*16
      |     msg_bottom = 'Real';
      |     label_out = sprintf('[%dx16-bit]',NumSample);
      | 
      | end
      | 
      | ReqBitWidth =  num2str(BitWidth);
      | fprintf('Channel \n Unpack \n ')
      | %text(0.50, 0.50, 'AXI4 Read', 'horizontalAlignment', 'center');
      | %color('blue');
      | %text(0.97, 0.87,'ALTERASOC', 'horizontalAlignment', 'right');
      | 
      | label_in = sprintf('[%d-bit]',BitWidth);
      | 
      | port_label('input',1,sprintf('DataIn \n%s',label_in))
      | port_label('output',1,sprintf('DataOut \n%s',label_out))
      | 
      | 
      | color('red');
      | text(0.15, 0.15,msg_bottom, 'horizontalAlignment', 'center')
  Time Scope : Scope  NumInputPorts=2
  wires:
  Subsystem1/1(Out1) -> Time Scope/1
  Tdata/1 -> Subsystem1/1(In1)
  Valid/1 -> Time Scope/2

== system SimplePulseGenerator_4x4_HDL_IQ/ADC_Triggered_Data_Capture/EnableConsecutiveFrames/sr_latch ==
  S : Inport
  R : Inport  Port=2
  Logical Operator1 : Logic  IconShape=distinctive  AllPortsSameDT=off  OutDataTypeStr=boolean
  Logical Operator2 : Logic  Operator=NOT  IconShape=distinctive  AllPortsSameDT=off  OutDataTypeStr=boolean
  Logical Operator9 : Logic  Operator=OR  IconShape=distinctive  AllPortsSameDT=off  OutDataTypeStr=boolean
  Unit Delay1 : UnitDelay  SampleTime=-1  HasFrameUpgradeWarning=on
  Q : Outport  VectorParamsAs1DForOutWhenUnconnected=off
  wires:
  S/1 -> Logical Operator9/1
  R/1 -> Logical Operator2/1
  Logical Operator2/1 -> Logical Operator1/1
  Unit Delay1/1 -> Logical Operator1/2, Q/1
  Logical Operator9/1 -> Unit Delay1/1
  Logical Operator1/1 -> Logical Operator9/2

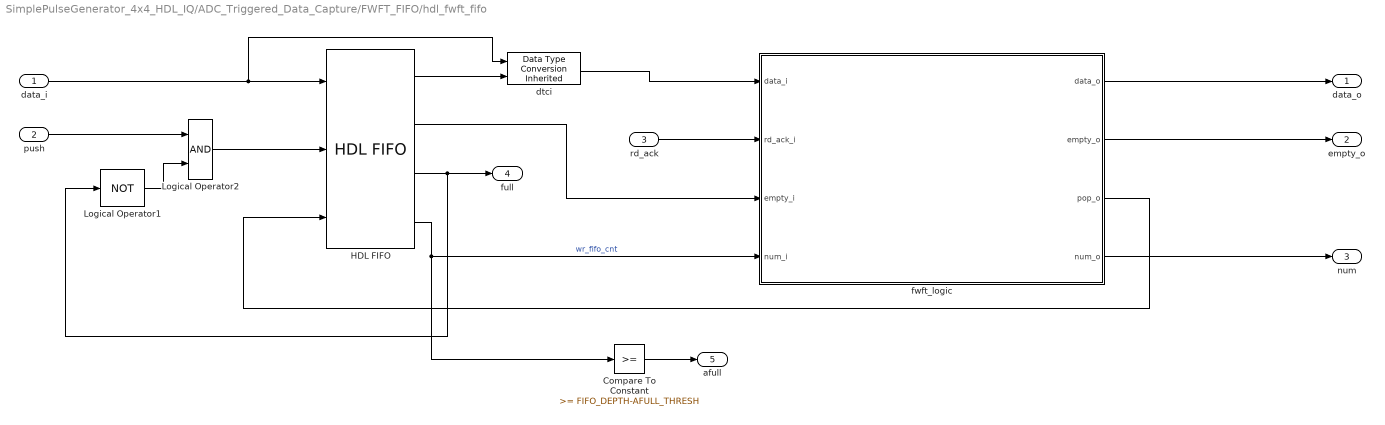
== system SimplePulseGenerator_4x4_HDL_IQ/ADC_Triggered_Data_Capture/FWFT_FIFO/hdl_fwft_fifo ==
  data_i : Inport
  push : Inport  Port=2
  rd_ack : Inport  Port=3
  Compare To Constant : simulink/Logic and Bit Operations/Compare To Constant  relop=>=  const=FIFO_DEPTH-AFULL_THRESH  OutDataTypeStr=boolean
  HDL FIFO : hdlsllib/HDL RAMs/HDL FIFO  fifo_size=FIFO_DEPTH  mode=Classic  ratio=1  push_msg=Error  pop_msg=Ignore  show_empty=on  show_full=on  show_num=on  LabelModeActiveChoice_Mode=Classic
      settings: SourceProductName=HDL Coder  SourceProductBaseCode=HD
  Logical Operator1 : Logic  Operator=NOT  IconShape=distinctive  AllPortsSameDT=off  OutDataTypeStr=boolean
  Logical Operator2 : Logic  IconShape=distinctive  AllPortsSameDT=off  OutDataTypeStr=boolean
  dtci : simulink/Signal Attributes/Data Type Conversion Inherited  ConvertRealWorld=Real World Value  DoSatur=off
      settings: SourceProductName=Simulink  SourceProductBaseCode=SL
  fwft_logic : Subsystem
  data_o : Outport  VectorParamsAs1DForOutWhenUnconnected=off
  empty_o : Outport  Port=2  VectorParamsAs1DForOutWhenUnconnected=off
  num : Outport  Port=3  VectorParamsAs1DForOutWhenUnconnected=off
  full : Outport  Port=4  VectorParamsAs1DForOutWhenUnconnected=off
  afull : Outport  Port=5  VectorParamsAs1DForOutWhenUnconnected=off
  wires:
  Compare To Constant/1 -> afull/1
  fwft_logic/1(data_o) -> data_o/1
  HDL FIFO/2 -> fwft_logic/3(empty_i)
  rd_ack/1 -> fwft_logic/2(rd_ack_i)
  fwft_logic/2(empty_o) -> empty_o/1
  data_i/1 -> dtci/1, HDL FIFO/1
  fwft_logic/3(pop_o) -> HDL FIFO/3
  push/1 -> Logical Operator2/1
  Logical Operator2/1 -> HDL FIFO/2
  Logical Operator1/1 -> Logical Operator2/2
  HDL FIFO/1 -> dtci/2
  dtci/1 -> fwft_logic/1(data_i)
  HDL FIFO/3 -> Logical Operator1/1, full/1
  HDL FIFO/4 -> Compare To Constant/1, fwft_logic/4(num_i)  "wr_fifo_cnt"
  fwft_logic/4(num_o) -> num/1

== system SimplePulseGenerator_4x4_HDL_IQ/ADC_Triggered_Data_Capture/NCO_Transmit/Subsystem4 ==
  Sample1 : Inport
  Sample2 : Inport  Port=2
  Sample3 : Inport  Port=3
  Sample4 : Inport  Port=4
  GainScale : Inport  Port=5
  Bit Concat : hdlsllib/Logic and Bit Operations/Bit Concat  numInputs=4
      settings: SourceProductName=HDL Coder  SourceProductBaseCode=HD
  Bit Concat1 : hdlsllib/Logic and Bit Operations/Bit Concat  numInputs=4
      settings: SourceProductName=HDL Coder  SourceProductBaseCode=HD
  Subsystem : Subsystem
  I_Samples : Outport  VectorParamsAs1DForOutWhenUnconnected=off
  Q_Samples : Outport  Port=2  VectorParamsAs1DForOutWhenUnconnected=off
  wires:
  Sample4/1 -> Subsystem/4(In4)
  Bit Concat/1 -> I_Samples/1
  Sample3/1 -> Subsystem/3(In3)
  Sample1/1 -> Subsystem/1(In1)
  Sample2/1 -> Subsystem/2(In2)
  GainScale/1 -> Subsystem/5(Scale)
  Subsystem/1(Sample1_I) -> Bit Concat/4
  Subsystem/3(Sample2_I) -> Bit Concat/3
  Subsystem/5(Sample3_I) -> Bit Concat/2
  Subsystem/7(Sample4_I) -> Bit Concat/1
  Subsystem/8(Sample4_Q) -> Bit Concat1/1
  Subsystem/6(Sample3_Q) -> Bit Concat1/2
  Subsystem/4(Sample2_Q) -> Bit Concat1/3
  Subsystem/2(Sample1_Q) -> Bit Concat1/4
  Bit Concat1/1 -> Q_Samples/1

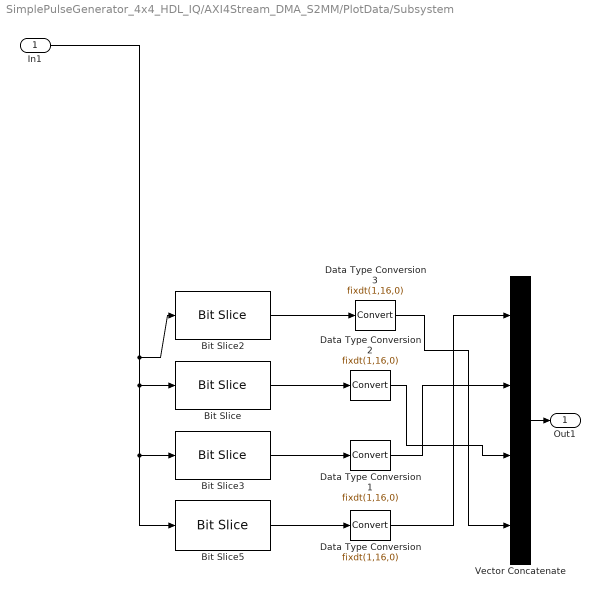
== system SimplePulseGenerator_4x4_HDL_IQ/AXI4Stream_DMA_S2MM/PlotData/Subsystem ==
  In1 : Inport
  Bit Slice : hdlsllib/Logic and Bit Operations/Bit Slice  lidx=47  ridx=32
  Bit Slice2 : hdlsllib/Logic and Bit Operations/Bit Slice  lidx=63  ridx=48
  Bit Slice3 : hdlsllib/Logic and Bit Operations/Bit Slice  lidx=31  ridx=16
  Bit Slice5 : hdlsllib/Logic and Bit Operations/Bit Slice  lidx=15  ridx=0
  Data Type Conversion{,1..3} (4 alike) : DataTypeConversion  OutDataTypeStr=fixdt(1,16,0)  ConvertRealWorld=Stored Integer (SI)
  Vector Concatenate : Concatenate  NumInputs=4  Mode=Multidimensional array
  Out1 : Outport  VectorParamsAs1DForOutWhenUnconnected=off
  wires:
  Data Type Conversion2/1 -> Vector Concatenate/3
  Bit Slice3/1 -> Data Type Conversion1/1
  Bit Slice2/1 -> Data Type Conversion3/1
  Data Type Conversion3/1 -> Vector Concatenate/4
  In1/1 -> Bit Slice2/1, Bit Slice3/1, Bit Slice5/1, Bit Slice/1
  Data Type Conversion1/1 -> Vector Concatenate/2
  Bit Slice/1 -> Data Type Conversion2/1
  Bit Slice5/1 -> Data Type Conversion/1
  Data Type Conversion/1 -> Vector Concatenate/1
  Vector Concatenate/1 -> Out1/1

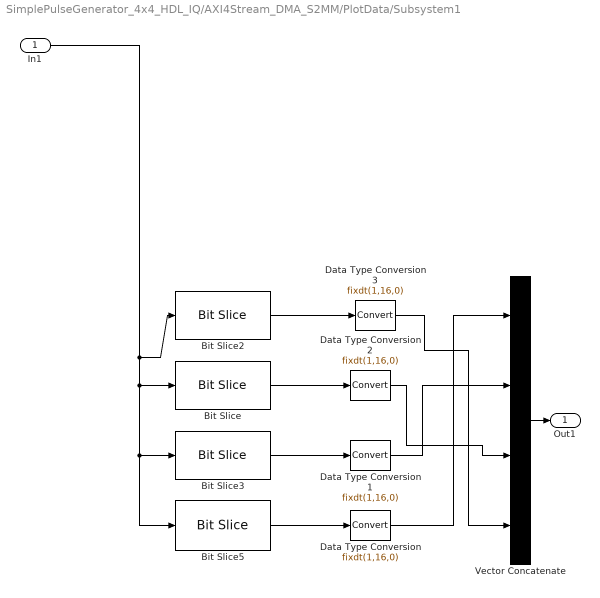
== system SimplePulseGenerator_4x4_HDL_IQ/AXI4Stream_DMA_S2MM/PlotData/Subsystem1 ==
  In1 : Inport
  Bit Slice : hdlsllib/Logic and Bit Operations/Bit Slice  lidx=47  ridx=32
  Bit Slice2 : hdlsllib/Logic and Bit Operations/Bit Slice  lidx=63  ridx=48
  Bit Slice3 : hdlsllib/Logic and Bit Operations/Bit Slice  lidx=31  ridx=16
  Bit Slice5 : hdlsllib/Logic and Bit Operations/Bit Slice  lidx=15  ridx=0
  Data Type Conversion{,1..3} (4 alike) : DataTypeConversion  OutDataTypeStr=fixdt(1,16,0)  ConvertRealWorld=Stored Integer (SI)
  Vector Concatenate : Concatenate  NumInputs=4  Mode=Multidimensional array
  Out1 : Outport  VectorParamsAs1DForOutWhenUnconnected=off
  wires:
  Vector Concatenate/1 -> Out1/1
  Data Type Conversion/1 -> Vector Concatenate/1
  Bit Slice5/1 -> Data Type Conversion/1
  Bit Slice/1 -> Data Type Conversion2/1
  Data Type Conversion1/1 -> Vector Concatenate/2
  In1/1 -> Bit Slice/1, Bit Slice5/1, Bit Slice3/1, Bit Slice2/1
  Data Type Conversion3/1 -> Vector Concatenate/4
  Bit Slice2/1 -> Data Type Conversion3/1
  Bit Slice3/1 -> Data Type Conversion1/1
  Data Type Conversion2/1 -> Vector Concatenate/3

== system SimplePulseGenerator_4x4_HDL_IQ/AXI4Stream_DMA_S2MM/Subsystem2/Subsystem1 ==
  In1 : Inport
  Constant6 : Constant  OutDataTypeStr=int16  SampleTime=-1
  FixPt Data Type Propagation : simulink/Signal Attributes/Data Type Propagation  PropDataType=sfix(16)  IfRefDouble=double  IfRefSingle=single  IsSigned=IsSigned1  NumBitsBase=NumBits1  NumBitsMult=1  NumBitsAdd=0  NumBitsAllowFinal=reqBitWidth  PropScaling=2^-10  ValuesUsedBestPrec=[5 -7]  SlopeBase=Slope1  SlopeMult=1  SlopeAdd=0  BiasBase=Bias1  BiasMult=1  BiasAdd=0
      settings: SourceProductName=Simulink  SourceProductBaseCode=SL
  MATLAB Function : MATLAB Function  TreatAsAtomicUnit=on
  Signal Specification1 : SignalSpecification  Dimensions=[samplesPerClock 1]
  Out1 : Outport  VectorParamsAs1DForOutWhenUnconnected=off
  wires:
  MATLAB Function/1(vector_out) -> Signal Specification1/1
  Constant6/1 -> FixPt Data Type Propagation/2
  In1/1 -> FixPt Data Type Propagation/1, FixPt Data Type Propagation/3, MATLAB Function/1(packed_in)
  Signal Specification1/1 -> Out1/1
